simulink model "test_adc083000x2"  (Simulink 7.4)
settings: Solver=ode45  StartTime=0.0  StopTime=100  RelTol=1e-3
libraries: isi_correlator_lib x5, xbsIndex_r4 x4, xps_library x4
settings Model: Creator=wjm  LastModifiedBy=wjm
settings OptimizationCC: InitFltsAndDblsToZero=on

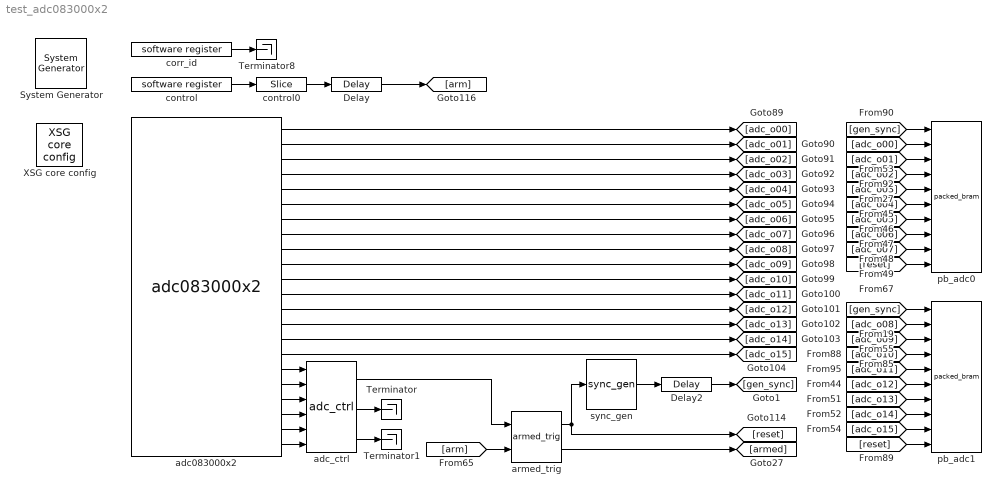
== system test_adc083000x2 ==
  " System Generator" : xbsIndex_r4/ System Generator  Tag=genX  SystemSampleTime=-1  xilinxfamily=virtex5  part=xc5vsx95t  speed=-1  package=ff1136  synthesis_tool=XST  clock_wrapper=Clock Enables  directory=./test_adc083000x2/sysgen  testbench=off  simulink_period=1  sysclk_period=2.6667  dcm_input_clock_period=100  incr_netlist=off  trim_vbits=Everywhere in SubSystem  dbl_ovrd=According to Block Masks  core_generation=According to Block Masks  run_coregen=off  deprecated_control=off  eval_field=0  block_type=sysgen
      settings: block_version=10.1.3
  Delay : xbsIndex_r4/Delay  en=off  latency=1  dbl_ovrd=off  reg_retiming=on  block_type=delay
      settings: block_version=11.3
  Delay2 : xbsIndex_r4/Delay  en=off  latency=1  dbl_ovrd=off  reg_retiming=on  block_type=delay
      settings: block_version=11.3
  Terminator : Terminator
  Terminator1 : Terminator
  Terminator8 : Terminator
  XSG core config : xps_library/XSG core config  Tag=xps:xsg  SystemSampleTime=-1  hw_sys=ROACH:sx95t  ibob_linux=off  clk_src=adc0_clk  iBOB_clk_src=sys_clk  BEE2_ctrl_clk_src=sys_clk  BEE2_usr_clk_src=sys_clk  ROACH_clk_src=adc0_clk  CORR_clk_src=sys_clk  gpio_clk_io_group=iBOB:sma  gpio_clk_bit_index=0  clk_rate=200  sample_period=1  synthesis_tool=XST  mpc_type=powerpc440_ext
  adc083000x2 : xps_library/adc083000x2  Tag=xps:adc083000x2  SystemSampleTime=-1  use_adc0=on  use_adc1=on  demux_adc=off  clock_sync=on  verbose=off  using_ctrl=off  adc_clk_rate=800  sample_period=1  bit_width=8
  adc_ctrl : isi_correlator_lib/adc_ctrl  SystemSampleTime=-1
  armed_trig : isi_correlator_lib/armed_trig  SystemSampleTime=-1
  control : xps_library/software register  Tag=xps:sw_reg  SystemSampleTime=-1  io_dir=From Processor  arith_type=Unsigned  bitwidth=32  bin_pt=0  sample_period=1  gw_name=test_adc083000x2_control_user_data_out
  control0 : xbsIndex_r4/Slice  nbits=1  boolean_output=on  mode=Lower Bit Location + Width  bit1=0  base1=MSB of Input  bit0=0  base0=LSB of Input  dbl_ovrd=off  block_type=slice
      settings: infoedit="Extracts a given range of bits from each input sample and presents it at the output.  The output type is ordinarily unsigned with binary point at zero, but can be Boolean when the slice is one bit wide.<P><P>Hardware notes: In hardware this block costs nothing."  block_version=10.1.3
  corr_id : xps_library/software register  Tag=xps:sw_reg  SystemSampleTime=-1  io_dir=From Processor  arith_type=Unsigned  bitwidth=32  bin_pt=0  sample_period=1  gw_name=test_adc083000x2_corr_id_user_data_out
  pb_adc0 : isi_correlator_lib/packed_bram  SystemSampleTime=-1  window_length=16  bit_width=8  fanin_latency=3
      settings: AttributesFormatString=size = 512B
  pb_adc1 : isi_correlator_lib/packed_bram  SystemSampleTime=-1  window_length=16  bit_width=8  fanin_latency=3
      settings: AttributesFormatString=size = 512B
  sync_gen : isi_correlator_lib/sync_gen  SystemSampleTime=-1
  wires:
  adc083000x2/17 -> adc_ctrl/1
  adc083000x2/18 -> adc_ctrl/2
  adc083000x2/19 -> adc_ctrl/3
  adc083000x2/20 -> adc_ctrl/4
  adc083000x2/21 -> adc_ctrl/5
  control0/1 -> Delay/1
  adc083000x2/22 -> adc_ctrl/6
  adc_ctrl/2 -> Terminator/1
  adc_ctrl/3 -> Terminator1/1
  [arm] -> armed_trig/2
  armed_trig/2 -> [armed]
  armed_trig/1 -> sync_gen/1, [reset]
  control/1 -> control0/1
  Delay/1 -> [arm]
  adc_ctrl/1 -> armed_trig/1
  sync_gen/1 -> Delay2/1
  adc083000x2/1 -> [adc_o00]
  adc083000x2/2 -> [adc_o01]
  adc083000x2/3 -> [adc_o02]
  adc083000x2/4 -> [adc_o03]
  adc083000x2/5 -> [adc_o04]
  adc083000x2/6 -> [adc_o05]
  adc083000x2/7 -> [adc_o06]
  adc083000x2/8 -> [adc_o07]
  adc083000x2/9 -> [adc_o08]
  adc083000x2/10 -> [adc_o09]
  adc083000x2/11 -> [adc_o10]
  adc083000x2/12 -> [adc_o11]
  adc083000x2/13 -> [adc_o12]
  adc083000x2/14 -> [adc_o13]
  adc083000x2/15 -> [adc_o14]
  adc083000x2/16 -> [adc_o15]
  [gen_sync] -> pb_adc0/1
  [adc_o00] -> pb_adc0/2
  [adc_o01] -> pb_adc0/3
  [adc_o02] -> pb_adc0/4
  [adc_o03] -> pb_adc0/5
  [adc_o04] -> pb_adc0/6
  [adc_o05] -> pb_adc0/7
  [adc_o06] -> pb_adc0/8
  [adc_o07] -> pb_adc0/9
  [reset] -> pb_adc0/10
  [gen_sync] -> pb_adc1/1
  [adc_o08] -> pb_adc1/2
  [adc_o09] -> pb_adc1/3
  [adc_o10] -> pb_adc1/4
  [adc_o11] -> pb_adc1/5
  [adc_o12] -> pb_adc1/6
  [adc_o13] -> pb_adc1/7
  [adc_o14] -> pb_adc1/8
  [adc_o15] -> pb_adc1/9
  [reset] -> pb_adc1/10
  Delay2/1 -> [gen_sync]
  corr_id/1 -> Terminator8/1
